simulink model "trajectoryGenerator"  (R2023b)
settings: Solver=VariableStepAuto  StartTime=0.0  StopTime=300  RelTol=1e-3
undefined symbols (not defined in the file): Prepocess, sgn
settings Model: Creator=daisy  LastModifiedBy=daisy

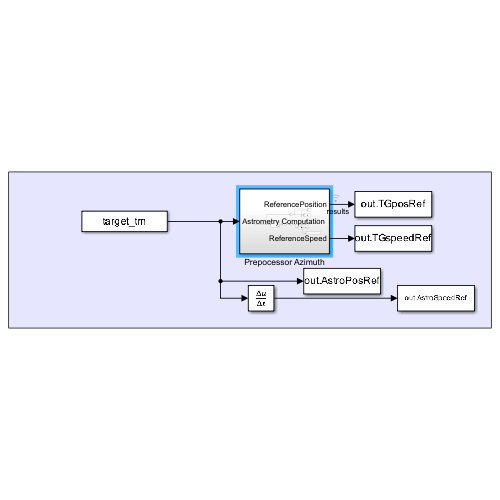
[thumbnail: Simulink's stored preview of the top-level diagram]
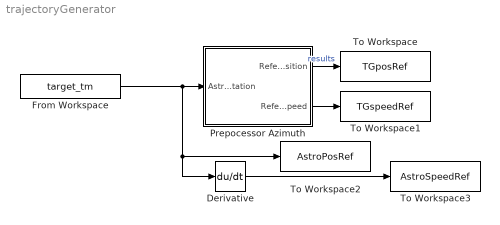
== system trajectoryGenerator ==
  Derivative : Derivative
  From Workspace : FromWorkspace  VariableName=target_tm
  Prepocessor Azimuth : Subsystem
  To Workspace : ToWorkspace  VariableName=TGposRef  SaveFormat=Timeseries  SampleTime=-1
  To Workspace1 : ToWorkspace  VariableName=TGspeedRef  SaveFormat=Timeseries  SampleTime=-1
  To Workspace2 : ToWorkspace  VariableName=AstroPosRef  SaveFormat=Timeseries  SampleTime=-1
  To Workspace3 : ToWorkspace  VariableName=AstroSpeedRef  SaveFormat=Timeseries  SampleTime=-1
  wires:
  Prepocessor Azimuth/1(ReferencePosition) -> To Workspace/1  "results"
  From Workspace/1 -> To Workspace2/1, Derivative/1, Prepocessor Azimuth/1(Astrometry Computation)
  Prepocessor Azimuth/2(ReferenceSpeed) -> To Workspace1/1
  Derivative/1 -> To Workspace3/1

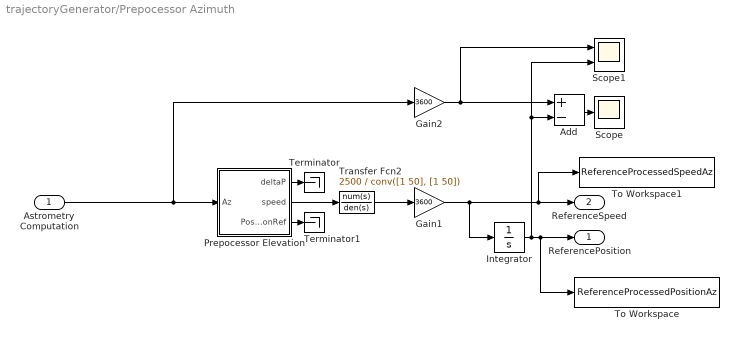
== system trajectoryGenerator/Prepocessor Azimuth ==
  Astrometry Computation : Inport
  Add : Sum  Inputs=+-
  Gain1 : Gain  Gain=3600
  Gain2 : Gain  Gain=3600
  Integrator : Integrator  InitialCondition=Prepocess.p0az*3600
  Prepocessor Elevation : Subsystem  TreatAsAtomicUnit=on  SystemSampleTime=Prepocess.Ts
  Scope : Scope
  Scope1 : Scope  NumInputPorts=2
  Terminator : Terminator
  Terminator1 : Terminator
  To Workspace : ToWorkspace  VariableName=ReferenceProcessedPositionAz  SaveFormat=Timeseries  SampleTime=-1
  To Workspace1 : ToWorkspace  VariableName=ReferenceProcessedSpeedAz  SaveFormat=Timeseries  SampleTime=-1
  Transfer Fcn2 : TransferFcn  Numerator=2500  Denominator=conv([1 50], [1 50])
  ReferencePosition : Outport
  ReferenceSpeed : Outport  Port=2
  wires:
  Gain2/1 -> Scope1/1, Add/1
  Add/1 -> Scope/1
  Gain1/1 -> Integrator/1, ReferenceSpeed/1, To Workspace1/1
  Transfer Fcn2/1 -> Gain1/1
  Prepocessor Elevation/3(PositionRef) -> Terminator1/1
  Integrator/1 -> ReferencePosition/1, To Workspace/1, Add/2, Scope1/2
  Prepocessor Elevation/1(deltaP) -> Terminator/1
  Prepocessor Elevation/2(speed) -> Transfer Fcn2/1
  Astrometry Computation/1 -> Prepocessor Elevation/1(Az), Gain2/1

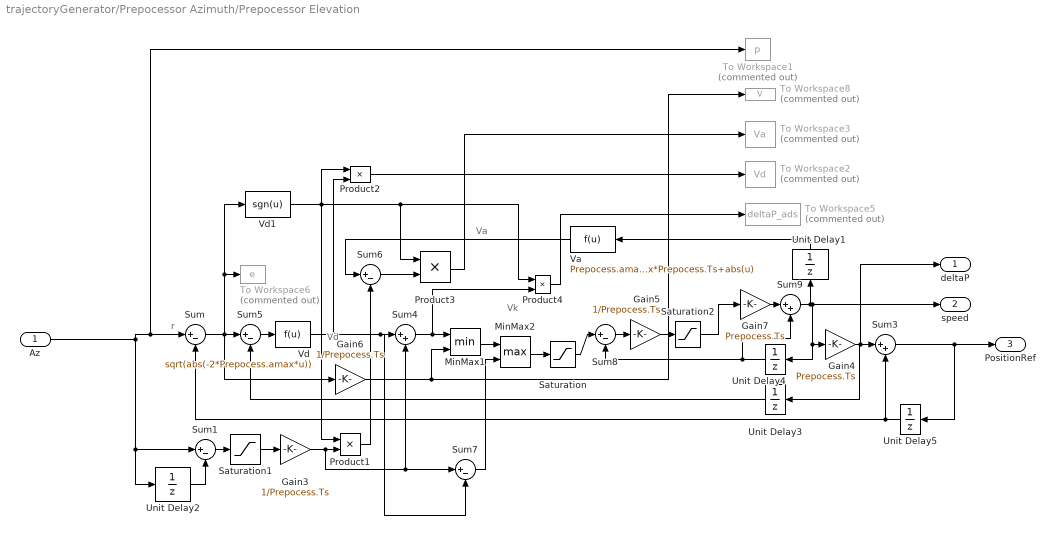
== system trajectoryGenerator/Prepocessor Azimuth/Prepocessor Elevation ==
  note: r
  note: Vk
  note: Va
  note: Vd
  Az : Inport
  Gain3 : Gain  Gain=1/Prepocess.Ts
  Gain4 : Gain  Gain=Prepocess.Ts
  Gain5 : Gain  Gain=1/Prepocess.Ts
  Gain6 : Gain  Gain=1/Prepocess.Ts
  Gain7 : Gain  Gain=Prepocess.Ts
  MinMax1 : MinMax  Inputs=2
  MinMax2 : MinMax  Function=max  Inputs=2
  Product{1..4} (4 alike) : Product
  Saturation : Saturate  UpperLimit=Prepocess.vmax  LowerLimit=-Prepocess.vmax
  Saturation1 : Saturate  UpperLimit=Prepocess.vmax*Prepocess.Ts  LowerLimit=-Prepocess.vmax*Prepocess.Ts
  Saturation2 : Saturate  UpperLimit=Prepocess.amax  LowerLimit=-Prepocess.amax
  Sum{,1,5..8} (6 alike) : Sum  Inputs=|+-
  Sum3 : Sum  Inputs=|++
  Sum4 : Sum  Inputs=|++
  Sum9 : Sum  Inputs=|++
  To Workspace1 : ToWorkspace  Commented=on  VariableName=p  SampleTime=-1
  To Workspace2 : ToWorkspace  Commented=on  VariableName=Vd  SampleTime=-1
  To Workspace3 : ToWorkspace  Commented=on  VariableName=Va  SampleTime=-1
  To Workspace5 : ToWorkspace  Commented=on  VariableName=deltaP_ads  SampleTime=-1
  To Workspace6 : ToWorkspace  Commented=on  VariableName=e  SampleTime=-1
  To Workspace8 : ToWorkspace  Commented=on  VariableName=V  SampleTime=-1
  Unit Delay{1..4} (4 alike) : UnitDelay  SampleTime=-1  HasFrameUpgradeWarning=on
  Unit Delay5 : UnitDelay  InitialCondition=Prepocess.p0az  SampleTime=-1  HasFrameUpgradeWarning=on
  Va : Fcn  Expr=Prepocess.amax*Prepocess.Ts+abs(u)
  Vd : Fcn  Expr=sqrt(abs(-2*Prepocess.amax*u))
  Vd1 : Fcn  Expr=sgn(u)
  deltaP : Outport
  speed : Outport  Port=2
  PositionRef : Outport  Port=3
  wires:
  Sum3/1 -> PositionRef/1, Unit Delay5/1
  Gain5/1 -> Saturation2/1
  Unit Delay1/1 -> Va/1
  MinMax2/1 -> Saturation/1
  Sum5/1 -> Vd/1
  Sum8/1 -> Gain5/1
  Saturation/1 -> Sum8/1
  Saturation1/1 -> Gain3/1
  Sum6/1 -> Product3/2
  Gain3/1 -> Product1/2, Sum4/2, Sum7/1
  MinMax1/1 -> MinMax2/1
  Gain6/1 -> To Workspace8/1, MinMax1/2
  Unit Delay4/1 -> Sum9/2, Sum8/2
  Sum9/1 -> Unit Delay1/1, Gain4/1, Unit Delay4/1, speed/1
  Gain7/1 -> Sum9/1
  Unit Delay2/1 -> Sum1/2
  Sum/1 -> To Workspace6/1, Vd1/1, Gain6/1, Sum5/1
  Sum1/1 -> Saturation1/1
  Va/1 -> Sum6/1
  Sum7/1 -> MinMax2/2
  Saturation2/1 -> Gain7/1
  Vd1/1 -> Product3/1, Product4/1, Product1/1, Product2/1
  Gain4/1 -> Unit Delay3/1, Sum3/1, deltaP/1
  Product1/1 -> Sum6/2
  Unit Delay3/1 -> Sum5/2
  Sum4/1 -> MinMax1/1, Product4/2
  Vd/1 -> Sum4/1, Sum7/2, Product2/2
  Product3/1 -> To Workspace3/1
  Product2/1 -> To Workspace2/1
  Az/1 -> To Workspace1/1, Sum/1, Sum1/1, Unit Delay2/1
  Product4/1 -> To Workspace5/1
  Unit Delay5/1 -> Sum3/2, Sum/2
